simulink model "sampleModel1422"  (R2023a)
settings: Solver=VariableStepAuto  StartTime=0.0  StopTime=10.0  RelTol=1e-3
libraries: simulink x2, hdlsllib x2
settings Model: Creator=user1  LastModifiedBy=user1

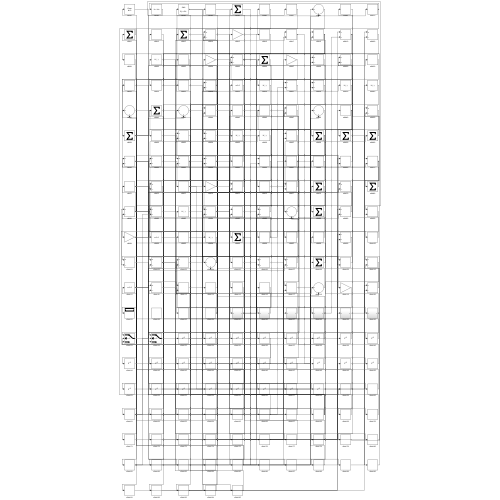
[thumbnail: Simulink's stored preview of the top-level diagram]
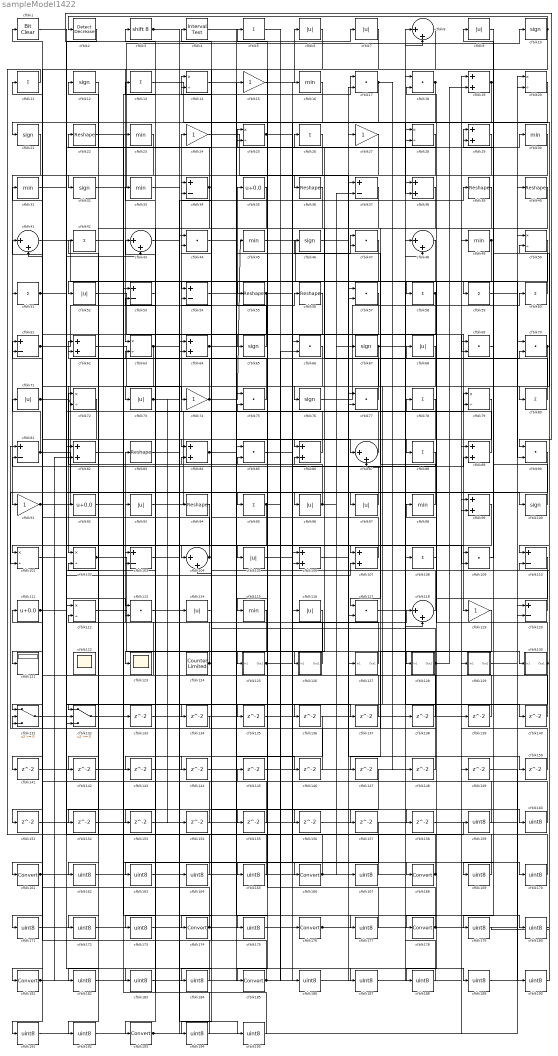
== system sampleModel1422 ==
  cfblk1 : simulink/Logic and Bit Operations/Bit Clear  iBit=0
      settings: LibrarySourceBlock=|
      | hdlsllib/Logic and Bit
      | Operations/Bit Clear
  cfblk{10,12,21,32,46,65,67,76,100} (9 alike) : Signum
  cfblk{14,20,25,28,50,63,72,79,101..102,112} (11 alike) : Product  Inputs=*/  RndMeth=Zero  SaturateOnIntegerOverflow=on
  cfblk{34,37,53..54,61,81,103,110,120} (9 alike) : Sum  Inputs=+-
  cfblk{8,41,43,48,87,104,118} (7 alike) : Sum  Inputs=|++
  cfblk{6..7,9,52,68,71,73,93,96..97,105,114,116} (13 alike) : Abs  SaturateOnIntegerOverflow=off
  cfblk{19,29,38,62,64,82,84,86,89,99,106..107} (12 alike) : Sum
  cfblk{5,11,13,26,42,51,58..60,78,80,88,95,108} (14 alike) : Sum  Inputs=+
  cfblk{17..18,44,47,57,66,69..70,75,77,85,90,109,113,117} (15 alike) : DotProduct  OutDataTypeStr=Inherit: Inherit via internal rule
  cfblk111 : Bias  Bias=0.0  SaturateOnIntegerOverflow=off
  cfblk{16,23,30..31,33,45,49,98,115} (9 alike) : MinMax
  cfblk{15,24,27,74,91,119} (6 alike) : Gain
  cfblk121 : Display
  cfblk122 : Scope
      settings: Floating=on
  cfblk123 : Scope
  cfblk124 : hdlsllib/Sources/Counter Limited  uplimit=7  tsamp=-1
  cfblk125 : Subsystem
      settings: LibrarySourceBlock=|
      | hdlsllib/Ports &
      | Subsystems/Subsystem
  cfblk126 : Subsystem
      settings: LibrarySourceBlock=|
      | hdlsllib/Ports &
      | Subsystems/Subsystem
  cfblk127 : Subsystem
      settings: LibrarySourceBlock=|
      | hdlsllib/Ports &
      | Subsystems/Subsystem
  cfblk128 : Subsystem
      settings: LibrarySourceBlock=|
      | hdlsllib/Ports &
      | Subsystems/Subsystem
  cfblk129 : Subsystem
      settings: LibrarySourceBlock=|
      | hdlsllib/Ports &
      | Subsystems/Subsystem
  cfblk130 : Subsystem
      settings: LibrarySourceBlock=|
      | hdlsllib/Ports &
      | Subsystems/Subsystem
  cfblk131 : Switch  SaturateOnIntegerOverflow=off  InputSameDT=off
  cfblk132 : Switch  SaturateOnIntegerOverflow=off  InputSameDT=off
  cfblk{133..158} (26 alike) : Delay  SampleTime=1
  cfblk{159..160,162..165,167,169..173,175,177,179..180,182..184,186..192,194..195} (28 alike) : DataTypeConversion  OutDataTypeStr=uint8  SaturateOnIntegerOverflow=off  RndMeth=Floor
  cfblk{161,166,168,174,176,178,181,185,193} (9 alike) : DataTypeConversion  SaturateOnIntegerOverflow=off  RndMeth=Floor
  cfblk2 : simulink/Logic and Bit Operations/Detect Decrease  vinit=0.0  OutDataTypeStr=boolean
      settings: LibrarySourceBlock=|
      | hdlsllib/Logic and Bit
      | Operations/Detect
      | Decrease
  cfblk{22,36,39..40,55..56,83,94} (8 alike) : Reshape
  cfblk3 : ArithShift  BitShiftNumber=8
  cfblk35 : Bias  Bias=0.0  SaturateOnIntegerOverflow=off
  cfblk4 : hdlsllib/Logic and Bit Operations/Interval Test  IntervalClosedRight=on  uplimit=0.5  IntervalClosedLeft=on  lowlimit=-0.5  OutDataTypeStr=boolean
  cfblk92 : Bias  Bias=0.0  SaturateOnIntegerOverflow=off
  wires:
  cfblk87/1 -> cfblk24/1
  cfblk8/1 -> cfblk63/1
  cfblk58/1 -> cfblk101/1, cfblk97/1
  cfblk15/1 -> cfblk6/1
  cfblk95/1 -> cfblk104/1, cfblk186/1
  cfblk62/1 -> cfblk74/1
  cfblk68/1 -> cfblk132/1
  cfblk102/1 -> cfblk128/1(In1), cfblk177/1
  cfblk103/1 -> cfblk39/1
  cfblk63/1 -> cfblk102/1, cfblk70/2
  cfblk118/1 -> cfblk22/1
  cfblk60/1 -> cfblk36/1
  cfblk34/1 -> cfblk12/1, cfblk143/1
  cfblk10/1 -> cfblk2/1, cfblk184/1
  cfblk13/1 -> cfblk80/1
  cfblk61/1 -> cfblk56/1, cfblk109/2, cfblk187/1
  cfblk21/1 -> cfblk91/1
  cfblk2/1 -> cfblk90/1
  cfblk38/1 -> cfblk73/1
  cfblk52/1 -> cfblk119/1
  cfblk32/1 -> cfblk10/1
  cfblk17/1 -> cfblk52/1, cfblk148/1
  cfblk115/1 -> cfblk123/1
  cfblk28/1 -> cfblk185/1
  cfblk48/1 -> cfblk76/1
  cfblk27/1 -> cfblk174/1
  cfblk37/1 -> cfblk126/1(In1)
  cfblk114/1 -> cfblk4/1
  cfblk76/1 -> cfblk60/1
  cfblk130/1(Out1) -> cfblk25/1, cfblk132/3
  cfblk131/1 -> cfblk78/1
  cfblk59/1 -> cfblk90/2
  cfblk107/1 -> cfblk34/1
  cfblk29/1 -> cfblk32/1
  cfblk77/1 -> cfblk26/1
  cfblk109/1 -> cfblk29/1
  cfblk91/1 -> cfblk68/1, cfblk95/1
  cfblk96/1 -> cfblk72/1, cfblk67/1, cfblk86/2
  cfblk42/1 -> cfblk166/1
  cfblk112/1 -> cfblk130/1(In1)
  cfblk65/1 -> cfblk35/1
  cfblk57/1 -> cfblk161/1
  cfblk41/1 -> cfblk70/1
  cfblk18/1 -> cfblk38/2, cfblk106/2, cfblk172/1
  cfblk45/1 -> cfblk108/1
  cfblk23/1 -> cfblk181/1
  cfblk100/1 -> cfblk9/1
  cfblk64/1 -> cfblk107/1, cfblk84/1, cfblk144/1
  cfblk30/1 -> cfblk131/1
  cfblk25/1 -> cfblk157/1, cfblk158/1
  cfblk46/1 -> cfblk127/1(In1)
  cfblk132/1 -> cfblk16/1
  cfblk53/1 -> cfblk193/1
  cfblk85/1 -> cfblk168/1
  cfblk71/1 -> cfblk72/2, cfblk79/2
  cfblk120/1 -> cfblk98/1
  cfblk128/1(Out1) -> cfblk131/2, cfblk19/2, cfblk84/2
  cfblk98/1 -> cfblk46/1
  cfblk75/1 -> cfblk62/1
  cfblk69/1 -> cfblk29/2
  cfblk3/1 -> cfblk109/1, cfblk189/1
  cfblk43/1 -> cfblk105/1
  cfblk67/1 -> cfblk140/1, cfblk141/1
  cfblk79/1 -> cfblk92/1
  cfblk26/1 -> cfblk51/1
  cfblk74/1 -> cfblk45/1, cfblk13/1
  cfblk55/1 -> cfblk69/2, cfblk152/1
  cfblk24/1 -> cfblk77/2
  cfblk70/1 -> cfblk179/1, cfblk192/1
  cfblk5/1 -> cfblk176/1
  cfblk88/1 -> cfblk81/2
  cfblk56/1 -> cfblk115/1
  cfblk93/1 -> cfblk25/2
  cfblk19/1 -> cfblk59/1, cfblk21/1
  cfblk49/1 -> cfblk88/1, cfblk86/1
  cfblk16/1 -> cfblk54/1
  cfblk40/1 -> cfblk117/1
  cfblk126/1(Out1) -> cfblk83/1
  cfblk84/1 -> cfblk47/1, cfblk180/1
  cfblk108/1 -> cfblk18/2
  cfblk129/1(Out1) -> cfblk120/1
  cfblk81/1 -> cfblk114/1, cfblk17/2, cfblk41/1, cfblk71/1, cfblk30/1
  cfblk1/1 -> cfblk100/1
  cfblk110/1 -> cfblk178/1
  cfblk97/1 -> cfblk14/1
  cfblk86/1 -> cfblk34/2
  cfblk127/1(Out1) -> cfblk93/1
  cfblk125/1(Out1) -> cfblk118/1, cfblk89/2, cfblk155/1
  cfblk39/1 -> cfblk125/1(In1)
  cfblk104/1 -> cfblk43/1, cfblk61/1
  cfblk51/1 -> cfblk113/1, cfblk7/1, cfblk43/2
  cfblk82/1 -> cfblk79/1
  cfblk89/1 -> cfblk3/1
  cfblk20/1 -> cfblk55/1
  cfblk73/1 -> cfblk64/2, cfblk154/1
  cfblk80/1 -> cfblk47/2
  cfblk36/1 -> cfblk65/1
  cfblk22/1 -> cfblk58/1
  cfblk124/1 -> cfblk14/2, cfblk112/2
  cfblk90/1 -> cfblk101/2
  cfblk92/1 -> cfblk17/1
  cfblk14/1 -> cfblk96/1
  cfblk117/1 -> cfblk48/1
  cfblk72/1 -> cfblk121/1
  cfblk44/1 -> cfblk87/1
  cfblk111/1 -> cfblk103/1, cfblk107/2, cfblk156/1
  cfblk133/1 -> cfblk44/1
  cfblk78/1 -> cfblk134/1
  cfblk134/1 -> cfblk131/3
  cfblk101/1 -> cfblk135/1
  cfblk135/1 -> cfblk19/1
  cfblk54/1 -> cfblk136/1
  cfblk105/1 -> cfblk137/1
  cfblk137/1 -> cfblk104/2
  cfblk138/1 -> cfblk1/1
  cfblk139/1 -> cfblk113/2
  cfblk140/1 -> cfblk62/2
  cfblk141/1 -> cfblk118/2
  cfblk12/1 -> cfblk142/1
  cfblk142/1 -> cfblk102/2
  cfblk143/1 -> cfblk8/2
  cfblk145/1 -> cfblk77/1
  cfblk4/1 -> cfblk146/1
  cfblk146/1 -> cfblk81/1
  cfblk119/1 -> cfblk147/1
  cfblk148/1 -> cfblk87/2
  cfblk106/1 -> cfblk150/1
  cfblk150/1 -> cfblk89/1
  cfblk6/1 -> cfblk151/1
  cfblk151/1 -> cfblk18/1
  cfblk152/1 -> cfblk20/1
  cfblk66/1 -> cfblk153/1
  cfblk153/1 -> cfblk64/1
  cfblk154/1 -> cfblk61/2
  cfblk155/1 -> cfblk103/2
  cfblk156/1 -> cfblk48/2
  cfblk158/1 -> cfblk120/2
  cfblk11/1 -> cfblk159/1
  cfblk159/1 -> cfblk75/1
  cfblk113/1 -> cfblk160/1
  cfblk160/1 -> cfblk11/1
  cfblk161/1 -> cfblk133/1, cfblk82/2, cfblk8/1
  cfblk35/1 -> cfblk162/1
  cfblk162/1 -> cfblk57/1
  cfblk157/1 -> cfblk163/1
  cfblk163/1 -> cfblk57/2
  cfblk33/1 -> cfblk164/1
  cfblk164/1 -> cfblk112/1
  cfblk116/1 -> cfblk165/1
  cfblk165/1 -> cfblk33/1
  cfblk166/1 -> cfblk145/1, cfblk37/2
  cfblk167/1 -> cfblk42/1
  cfblk168/1 -> cfblk75/2, cfblk82/1, cfblk63/2, cfblk44/2
  cfblk9/1 -> cfblk169/1
  cfblk169/1 -> cfblk85/1
  cfblk144/1 -> cfblk170/1
  cfblk170/1 -> cfblk85/2
  cfblk99/1 -> cfblk171/1
  cfblk171/1 -> cfblk117/2
  cfblk172/1 -> cfblk99/1
  cfblk136/1 -> cfblk173/1
  cfblk173/1 -> cfblk99/2
  cfblk174/1 -> cfblk41/2, cfblk40/1, cfblk116/1
  cfblk7/1 -> cfblk175/1
  cfblk175/1 -> cfblk27/1
  cfblk176/1 -> cfblk37/1, cfblk129/1(In1)
  cfblk177/1 -> cfblk5/1
  cfblk178/1 -> cfblk149/1, cfblk106/1
  cfblk179/1 -> cfblk110/1
  cfblk180/1 -> cfblk110/2
  cfblk181/1 -> cfblk167/1, cfblk132/2, cfblk66/1
  cfblk47/1 -> cfblk182/1
  cfblk182/1 -> cfblk23/1
  cfblk31/1 -> cfblk183/1
  cfblk183/1 -> cfblk15/1
  cfblk184/1 -> cfblk31/1
  cfblk185/1 -> cfblk139/1, cfblk138/1, cfblk66/2, cfblk111/1, cfblk54/2
  cfblk186/1 -> cfblk28/1
  cfblk187/1 -> cfblk28/2
  cfblk50/1 -> cfblk188/1
  cfblk188/1 -> cfblk38/1
  cfblk189/1 -> cfblk50/1
  cfblk149/1 -> cfblk190/1
  cfblk190/1 -> cfblk50/2
  cfblk94/1 -> cfblk191/1
  cfblk191/1 -> cfblk69/1
  cfblk192/1 -> cfblk94/1
  cfblk193/1 -> cfblk20/2, cfblk49/1
  cfblk147/1 -> cfblk194/1
  cfblk194/1 -> cfblk53/1
  cfblk83/1 -> cfblk195/1
  cfblk195/1 -> cfblk53/2

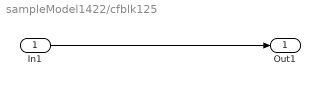
== system sampleModel1422/cfblk125 ==
  In1 : Inport
  Out1 : Outport
  wires:
  In1/1 -> Out1/1

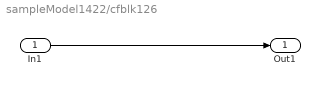
== system sampleModel1422/cfblk126 ==
  In1 : Inport
  Out1 : Outport
  wires:
  In1/1 -> Out1/1

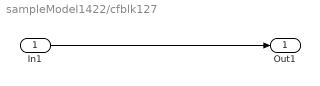
== system sampleModel1422/cfblk127 ==
  In1 : Inport
  Out1 : Outport
  wires:
  In1/1 -> Out1/1

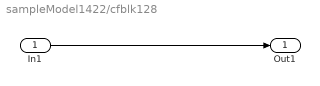
== system sampleModel1422/cfblk128 ==
  In1 : Inport
  Out1 : Outport
  wires:
  In1/1 -> Out1/1

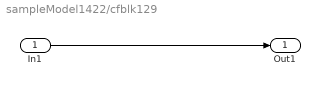
== system sampleModel1422/cfblk129 ==
  In1 : Inport
  Out1 : Outport
  wires:
  In1/1 -> Out1/1

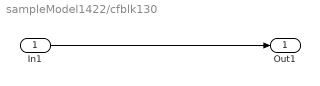
== system sampleModel1422/cfblk130 ==
  In1 : Inport
  Out1 : Outport
  wires:
  In1/1 -> Out1/1
